simulink model "sampleModel1694"  (R2023a)
settings: Solver=VariableStepAuto  StartTime=0.0  StopTime=10.0  RelTol=1e-3
libraries: hdlsllib x5, simulink x2
settings Model: Creator=user1  LastModifiedBy=user1

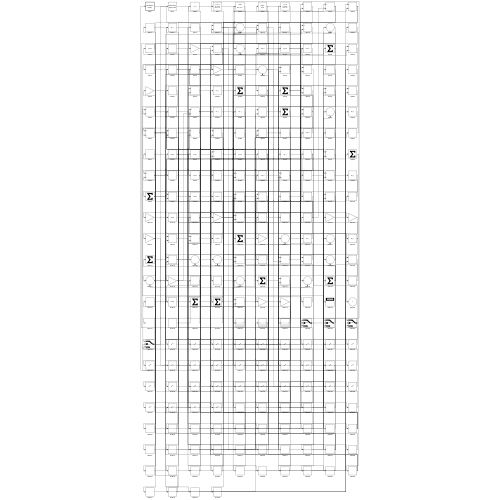
[thumbnail: Simulink's stored preview of the top-level diagram]
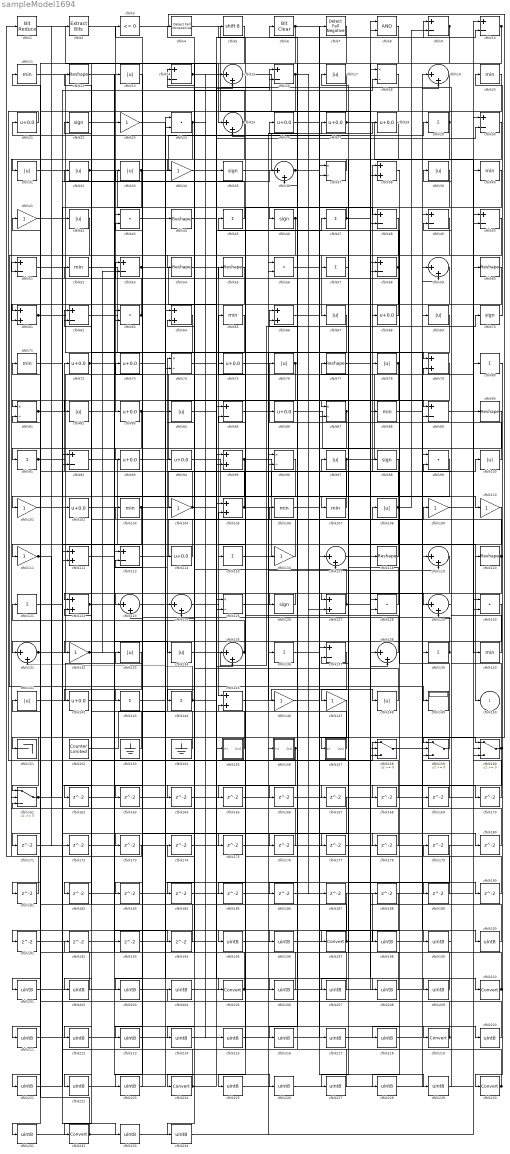
== system sampleModel1694 ==
  cfblk1 : hdlsllib/Logic and Bit Operations/Bit Reduce  mode=AND
  cfblk{9..10,14,16,30,48..51,53,58,62,85,89,92,113,137} (17 alike) : Sum  Inputs=+-
  cfblk{13,17,31..33,39,42,67,69,76,78,82,84,97,100,108,133..134,141,148} (20 alike) : Abs  SaturateOnIntegerOverflow=off
  cfblk{23,34,41,101,104,109..111,116,132,146..147} (12 alike) : Gain
  cfblk{21,26..28,68,72..73,75,83,86,93..94,102,114,142} (15 alike) : Bias  Bias=0.0  SaturateOnIntegerOverflow=off
  cfblk{11,20,40,52,65,71,88,103,106..107,140} (11 alike) : MinMax
  cfblk{38,61,64,66,79,95,105,112,122,127,145} (11 alike) : Sum
  cfblk{29,45,47,57,80,91,115,121,136,139,143..144} (12 alike) : Sum  Inputs=+
  cfblk{15,19,25,36,59,117,119,123..124,129,131,135,138} (13 alike) : Sum  Inputs=|++
  cfblk{12,44,54..55,60,77,90,118,120} (9 alike) : Reshape
  cfblk{18,37,74,81,87,96,125} (7 alike) : Product  Inputs=*/  RndMeth=Zero  SaturateOnIntegerOverflow=on
  cfblk{22,35,46,70,98,126} (6 alike) : Signum
  cfblk{24,43,56,63,99,128,130} (7 alike) : DotProduct  OutDataTypeStr=Inherit: Inherit via internal rule
  cfblk149 : Display
  cfblk151 : Terminator
  cfblk152 : hdlsllib/Sources/Counter Limited  uplimit=7  tsamp=-1
  cfblk153 : Ground
  cfblk154 : Ground
  cfblk155 : Subsystem
      settings: LibrarySourceBlock=|
      | hdlsllib/Ports &
      | Subsystems/Subsystem
  cfblk156 : Subsystem
      settings: LibrarySourceBlock=|
      | hdlsllib/Ports &
      | Subsystems/Subsystem
  cfblk157 : Subsystem
      settings: LibrarySourceBlock=|
      | hdlsllib/Ports &
      | Subsystems/Subsystem
  cfblk{158..161} (4 alike) : Switch  SaturateOnIntegerOverflow=off  InputSameDT=off
  cfblk{162..194} (33 alike) : Delay  SampleTime=1
  cfblk{195..196,198..204,206..209,211..218,220..223,225..229,231,233..234} (33 alike) : DataTypeConversion  OutDataTypeStr=uint8  SaturateOnIntegerOverflow=off  RndMeth=Floor
  cfblk{197,205,210,219,224,230,232} (7 alike) : DataTypeConversion  SaturateOnIntegerOverflow=off  RndMeth=Floor
  cfblk2 : simulink/Logic and Bit Operations/Extract Bits  bitsToExtract=Upper half  numBits=8  bitIdxRange=[0 7]  outScalingMode=Preserve fixed-point scaling
      settings: LibrarySourceBlock=|
      | hdlsllib/Logic and Bit
      | Operations/Extract Bits
  cfblk3 : hdlsllib/Logic and Bit Operations/Compare To Zero  relop=<=  OutDataTypeStr=boolean
  cfblk4 : hdlsllib/Logic and Bit Operations/Detect Fall Nonpositive  vinit=0  OutDataTypeStr=boolean
  cfblk5 : ArithShift  BitShiftNumber=8
  cfblk6 : simulink/Logic and Bit Operations/Bit Clear  iBit=0
      settings: LibrarySourceBlock=|
      | hdlsllib/Logic and Bit
      | Operations/Bit Clear
  cfblk7 : hdlsllib/Logic and Bit Operations/Detect Fall Negative  vinit=0  OutDataTypeStr=boolean
  cfblk8 : Logic  AllPortsSameDT=off  OutDataTypeStr=boolean
  cfblk150 : Outport  VectorParamsAs1DForOutWhenUnconnected=off
  wires:
  cfblk145/1 -> cfblk148/1
  cfblk105/1 -> cfblk72/1, cfblk107/1
  cfblk100/1 -> cfblk76/1
  cfblk134/1 -> cfblk70/1
  cfblk87/1 -> cfblk91/1, cfblk165/1
  cfblk42/1 -> cfblk149/1
  cfblk80/1 -> cfblk230/1
  cfblk113/1 -> cfblk108/1
  cfblk120/1 -> cfblk97/1, cfblk123/2
  cfblk61/1 -> cfblk136/1, cfblk16/2, cfblk233/1
  cfblk104/1 -> cfblk41/1, cfblk10/2, cfblk15/2, cfblk18/2
  cfblk11/1 -> cfblk138/1
  cfblk17/1 -> cfblk61/1
  cfblk6/1 -> cfblk214/1, cfblk229/1
  cfblk2/1 -> cfblk83/1
  cfblk108/1 -> cfblk12/1, cfblk9/2, cfblk127/1, cfblk55/1
  cfblk135/1 -> cfblk121/1, cfblk225/1
  cfblk69/1 -> cfblk157/1(In1)
  cfblk14/1 -> cfblk16/1, cfblk15/1, cfblk215/1
  cfblk128/1 -> cfblk21/1
  cfblk47/1 -> cfblk46/1, cfblk9/1, cfblk129/1
  cfblk137/1 -> cfblk147/1
  cfblk33/1 -> cfblk29/1, cfblk92/2, cfblk178/1
  cfblk131/1 -> cfblk38/1, cfblk36/1
  cfblk10/1 -> cfblk126/1, cfblk211/1
  cfblk54/1 -> cfblk145/1
  cfblk29/1 -> cfblk23/1, cfblk57/1
  cfblk31/1 -> cfblk113/1
  cfblk144/1 -> cfblk47/1, cfblk131/2
  cfblk130/1 -> cfblk232/1
  cfblk157/1(Out1) -> cfblk73/1
  cfblk20/1 -> cfblk123/1
  cfblk35/1 -> cfblk27/1
  cfblk155/1(Out1) -> cfblk74/1
  cfblk21/1 -> cfblk158/1
  cfblk18/1 -> cfblk101/1
  cfblk66/1 -> cfblk137/1
  cfblk41/1 -> cfblk102/1
  cfblk25/1 -> cfblk144/1, cfblk4/1
  cfblk91/1 -> cfblk65/1, cfblk164/1
  cfblk140/1 -> cfblk14/1
  cfblk37/1 -> cfblk31/1
  cfblk124/1 -> cfblk135/1
  cfblk7/1 -> cfblk25/1
  cfblk103/1 -> cfblk100/1, cfblk79/2, cfblk181/1
  cfblk107/1 -> cfblk66/1
  cfblk40/1 -> cfblk158/2
  cfblk93/1 -> cfblk8/1
  cfblk126/1 -> cfblk122/1
  cfblk123/1 -> cfblk44/1
  cfblk62/1 -> cfblk125/1
  cfblk50/1 -> cfblk224/1
  cfblk75/1 -> cfblk68/1
  cfblk83/1 -> cfblk111/1, cfblk7/1
  cfblk48/1 -> cfblk67/1
  cfblk46/1 -> cfblk196/1, cfblk231/1
  cfblk156/1(Out1) -> cfblk36/2, cfblk185/1
  cfblk13/1 -> cfblk143/1
  cfblk109/1 -> cfblk90/1
  cfblk43/1 -> cfblk205/1
  cfblk30/1 -> cfblk81/1
  cfblk129/1 -> cfblk39/1
  cfblk1/1 -> cfblk155/1(In1)
  cfblk111/1 -> cfblk171/1, cfblk172/1
  cfblk9/1 -> cfblk38/2, cfblk82/1
  cfblk89/1 -> cfblk60/1
  cfblk3/1 -> cfblk159/1
  cfblk24/1 -> cfblk51/2, cfblk35/1, cfblk182/1
  cfblk77/1 -> cfblk8/2
  cfblk85/1 -> cfblk119/2
  cfblk115/1 -> cfblk78/1
  cfblk86/1 -> cfblk118/1
  cfblk72/1 -> cfblk110/1, cfblk209/1
  cfblk160/1 -> cfblk129/2, cfblk218/1
  cfblk132/1 -> cfblk53/2, cfblk175/1
  cfblk53/1 -> cfblk125/2, cfblk79/1
  cfblk114/1 -> cfblk22/1
  cfblk23/1 -> cfblk48/1
  cfblk8/1 -> cfblk34/1
  cfblk121/1 -> cfblk42/1
  cfblk99/1 -> cfblk197/1
  cfblk136/1 -> cfblk160/1
  cfblk56/1 -> cfblk37/2
  cfblk118/1 -> cfblk85/2
  cfblk95/1 -> cfblk158/3, cfblk234/1
  cfblk45/1 -> cfblk32/1
  cfblk92/1 -> cfblk150/1
  cfblk158/1 -> cfblk69/1
  cfblk139/1 -> cfblk103/1, cfblk5/1
  cfblk58/1 -> cfblk17/1, cfblk61/2
  cfblk51/1 -> cfblk139/1
  cfblk63/1 -> cfblk11/1, cfblk93/1
  cfblk16/1 -> cfblk127/2, cfblk183/1
  cfblk67/1 -> cfblk132/1
  cfblk27/1 -> cfblk140/1, cfblk89/2
  cfblk152/1 -> cfblk74/2
  cfblk148/1 -> cfblk94/1
  cfblk28/1 -> cfblk151/1
  cfblk32/1 -> cfblk104/1, cfblk48/2
  cfblk125/1 -> cfblk28/1
  cfblk97/1 -> cfblk40/1, cfblk142/1
  cfblk127/1 -> cfblk64/2, cfblk109/1
  cfblk122/1 -> cfblk134/1, cfblk114/1
  cfblk4/1 -> cfblk98/1
  cfblk81/1 -> cfblk58/2, cfblk120/1
  cfblk82/1 -> cfblk13/1
  cfblk117/1 -> cfblk210/1
  cfblk52/1 -> cfblk146/1
  cfblk141/1 -> cfblk63/1
  cfblk70/1 -> cfblk20/1
  cfblk73/1 -> cfblk87/1
  cfblk94/1 -> cfblk116/1
  cfblk119/1 -> cfblk124/2
  cfblk112/1 -> cfblk219/1
  cfblk138/1 -> cfblk75/1
  cfblk68/1 -> cfblk3/1
  cfblk76/1 -> cfblk201/1, cfblk212/1
  cfblk15/1 -> cfblk128/1
  cfblk74/1 -> cfblk30/2
  cfblk39/1 -> cfblk115/1
  cfblk116/1 -> cfblk62/1
  cfblk161/1 -> cfblk2/1, cfblk170/1
  cfblk159/1 -> cfblk45/1
  cfblk5/1 -> cfblk54/1
  cfblk154/1 -> cfblk53/1
  cfblk78/1 -> cfblk128/2, cfblk131/1
  cfblk153/1 -> cfblk52/1
  cfblk147/1 -> cfblk161/1
  cfblk36/1 -> cfblk89/1, cfblk187/1
  cfblk64/1 -> cfblk162/1
  cfblk162/1 -> cfblk58/1
  cfblk65/1 -> cfblk163/1
  cfblk163/1 -> cfblk124/1
  cfblk164/1 -> cfblk87/2
  cfblk165/1 -> cfblk160/2
  cfblk71/1 -> cfblk166/1
  cfblk102/1 -> cfblk167/1
  cfblk34/1 -> cfblk168/1
  cfblk168/1 -> cfblk122/2
  cfblk169/1 -> cfblk159/2
  cfblk170/1 -> cfblk10/1
  cfblk171/1 -> cfblk135/2
  cfblk101/1 -> cfblk173/1
  cfblk173/1 -> cfblk1/1
  cfblk174/1 -> cfblk30/1
  cfblk175/1 -> cfblk37/1
  cfblk79/1 -> cfblk176/1
  cfblk176/1 -> cfblk95/1
  cfblk57/1 -> cfblk177/1
  cfblk177/1 -> cfblk137/2
  cfblk178/1 -> cfblk105/2
  cfblk84/1 -> cfblk180/1
  cfblk180/1 -> cfblk51/1
  cfblk181/1 -> cfblk161/2
  cfblk182/1 -> cfblk160/3
  cfblk183/1 -> cfblk138/2
  cfblk90/1 -> cfblk184/1
  cfblk184/1 -> cfblk14/2
  cfblk185/1 -> cfblk119/1
  cfblk60/1 -> cfblk186/1
  cfblk186/1 -> cfblk66/2
  cfblk26/1 -> cfblk189/1
  cfblk189/1 -> cfblk56/1
  cfblk143/1 -> cfblk190/1
  cfblk190/1 -> cfblk25/2
  cfblk98/1 -> cfblk191/1
  cfblk191/1 -> cfblk85/1
  cfblk192/1 -> cfblk63/2
  cfblk22/1 -> cfblk193/1
  cfblk193/1 -> cfblk113/2
  cfblk142/1 -> cfblk194/1
  cfblk194/1 -> cfblk81/2
  cfblk188/1 -> cfblk195/1
  cfblk195/1 -> cfblk159/3
  cfblk196/1 -> cfblk188/1
  cfblk197/1 -> cfblk169/1, cfblk62/2
  cfblk110/1 -> cfblk198/1
  cfblk198/1 -> cfblk99/1
  cfblk146/1 -> cfblk199/1
  cfblk199/1 -> cfblk99/2
  cfblk88/1 -> cfblk200/1
  cfblk200/1 -> cfblk18/1
  cfblk201/1 -> cfblk88/1
  cfblk59/1 -> cfblk202/1
  cfblk202/1 -> cfblk141/1
  cfblk167/1 -> cfblk203/1
  cfblk203/1 -> cfblk59/1
  cfblk204/1 -> cfblk59/2
  cfblk205/1 -> cfblk192/1, cfblk105/1
  cfblk44/1 -> cfblk206/1
  cfblk206/1 -> cfblk43/1
  cfblk179/1 -> cfblk207/1
  cfblk207/1 -> cfblk43/2
  cfblk106/1 -> cfblk208/1
  cfblk208/1 -> cfblk77/1
  cfblk209/1 -> cfblk106/1
  cfblk210/1 -> cfblk179/1, cfblk174/1, cfblk84/1, cfblk33/1
  cfblk211/1 -> cfblk117/1
  cfblk212/1 -> cfblk117/2
  cfblk96/1 -> cfblk213/1
  cfblk213/1 -> cfblk156/1(In1)
  cfblk214/1 -> cfblk96/1
  cfblk215/1 -> cfblk96/2
  cfblk19/1 -> cfblk216/1
  cfblk216/1 -> cfblk86/1
  cfblk166/1 -> cfblk217/1
  cfblk217/1 -> cfblk19/1
  cfblk218/1 -> cfblk19/2
  cfblk219/1 -> cfblk204/1, cfblk161/3, cfblk6/1
  cfblk12/1 -> cfblk220/1
  cfblk220/1 -> cfblk112/1
  cfblk187/1 -> cfblk221/1
  cfblk221/1 -> cfblk112/2
  cfblk133/1 -> cfblk222/1
  cfblk222/1 -> cfblk24/2
  cfblk55/1 -> cfblk223/1
  cfblk223/1 -> cfblk133/1
  cfblk224/1 -> cfblk95/2, cfblk64/1
  cfblk225/1 -> cfblk50/1
  cfblk172/1 -> cfblk226/1
  cfblk226/1 -> cfblk50/2
  cfblk49/1 -> cfblk227/1
  cfblk227/1 -> cfblk26/1
  cfblk38/1 -> cfblk228/1
  cfblk228/1 -> cfblk49/1
  cfblk229/1 -> cfblk49/2
  cfblk230/1 -> cfblk92/1, cfblk145/2, cfblk24/1
  cfblk231/1 -> cfblk80/1
  cfblk232/1 -> cfblk56/2, cfblk71/1
  cfblk233/1 -> cfblk130/1
  cfblk234/1 -> cfblk130/2

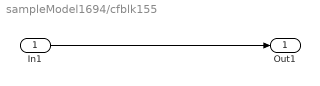
== system sampleModel1694/cfblk155 ==
  In1 : Inport
  Out1 : Outport
  wires:
  In1/1 -> Out1/1

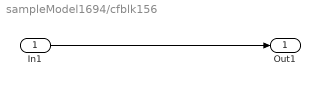
== system sampleModel1694/cfblk156 ==
  In1 : Inport
  Out1 : Outport
  wires:
  In1/1 -> Out1/1

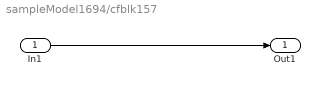
== system sampleModel1694/cfblk157 ==
  In1 : Inport
  Out1 : Outport
  wires:
  In1/1 -> Out1/1
